simulink model "case3"  (R2024b)
settings: Solver=FixedStepAuto  StartTime=0  StopTime=1  FixedStep=1e-7  RelTol=1e-3
values from neighbouring files (symbols this model uses):
  SG_D_1_D = 0.01056    [IEEE9_case_parameters.m]    (also in case1_parameters.m; case2_parameters.m; case3_parameters.m; case4_parameters.m)
  SG_D_1_EnableSaturation = 0    [IEEE9_case_parameters.m]    (also in case1_parameters.m; case2_parameters.m; case3_parameters.m; case4_parameters.m)
  SG_D_1_f0 = 60    [IEEE9_case_parameters.m]    (also in case1_parameters.m; case2_parameters.m; case3_parameters.m; case4_parameters.m)
  SG_D_1_H = 7.5    [IEEE9_case_parameters.m]    (also in case1_parameters.m; case2_parameters.m; case3_parameters.m; case4_parameters.m)
  SG_D_1_K_A = 20    [IEEE9_case_parameters.m]    (also in case1_parameters.m; case2_parameters.m; case3_parameters.m; case4_parameters.m)
  SG_D_1_K_E = 1.000000e+1    (= 10)    [IEEE9_case_parameters.m]    (also in case1_parameters.m; case2_parameters.m; case3_parameters.m; case4_parameters.m)
  SG_D_1_K_F = 2.363    [IEEE9_case_parameters.m]    (also in case1_parameters.m; case2_parameters.m; case3_parameters.m; case4_parameters.m)
  SG_D_1_K_s = 0.5    [IEEE9_case_parameters.m]    (also in case1_parameters.m = 5; case2_parameters.m = 5; case3_parameters.m = 5; case4_parameters.m = 5)
  SG_D_1_R_a = 0.001088    [IEEE9_case_parameters.m]    (also in case1_parameters.m; case2_parameters.m; case3_parameters.m; case4_parameters.m)
  SG_D_1_S_A = 1    [IEEE9_case_parameters.m]    (also in case1_parameters.m; case2_parameters.m; case3_parameters.m; case4_parameters.m)
  SG_D_1_S_B = 0.103    [IEEE9_case_parameters.m]    (also in case1_parameters.m; case2_parameters.m; case3_parameters.m; case4_parameters.m)
  SG_D_1_S_N = 10.659857    [IEEE9_case_parameters.m]    (also in case1_parameters.m; case2_parameters.m; case3_parameters.m; case4_parameters.m)
  SG_D_1_SpeedPara = 200    [IEEE9_case_parameters.m]    (also in case1_parameters.m; case2_parameters.m; case3_parameters.m; case4_parameters.m)
  SG_D_1_T_0 = 0.720173    [IEEE9_case_parameters.m]    (also in case1_parameters.m = 0.755522; case2_parameters.m = 0.808931; case3_parameters.m = 0.869402; case4_parameters.m = 0.729316)
  SG_D_1_T_1 = 0.3    [IEEE9_case_parameters.m]    (also in case1_parameters.m; case2_parameters.m; case3_parameters.m; case4_parameters.m)
  SG_D_1_T_2 = 0.05    [IEEE9_case_parameters.m]    (also in case1_parameters.m; case2_parameters.m; case3_parameters.m; case4_parameters.m)
  SG_D_1_T_3 = 0.02    [IEEE9_case_parameters.m]    (also in case1_parameters.m; case2_parameters.m; case3_parameters.m; case4_parameters.m)
  SG_D_1_T_4 = 0.005    [IEEE9_case_parameters.m]    (also in case1_parameters.m; case2_parameters.m; case3_parameters.m; case4_parameters.m)
  SG_D_1_T_A = 0.02    [IEEE9_case_parameters.m]    (also in case1_parameters.m; case2_parameters.m; case3_parameters.m; case4_parameters.m)
  SG_D_1_T_dd = 8.000000e+0    (= 8)    [IEEE9_case_parameters.m]    (also in case1_parameters.m; case2_parameters.m; case3_parameters.m; case4_parameters.m)
  SG_D_1_T_ddd = 0.04    [IEEE9_case_parameters.m]    (also in case1_parameters.m; case2_parameters.m; case3_parameters.m; case4_parameters.m)
  SG_D_1_T_E = 0.314    [IEEE9_case_parameters.m]    (also in case1_parameters.m; case2_parameters.m; case3_parameters.m; case4_parameters.m)
  SG_D_1_T_F = 0.35    [IEEE9_case_parameters.m]    (also in case1_parameters.m; case2_parameters.m; case3_parameters.m; case4_parameters.m)
  SG_D_1_T_qd = 0.8    [IEEE9_case_parameters.m]    (also in case1_parameters.m; case2_parameters.m; case3_parameters.m; case4_parameters.m)
  SG_D_1_T_qdd = 0.02    [IEEE9_case_parameters.m]    (also in case1_parameters.m; case2_parameters.m; case3_parameters.m; case4_parameters.m)
  SG_D_1_T_speed = 0.1    [IEEE9_case_parameters.m]    (also in case1_parameters.m = 200; case2_parameters.m = 200; case3_parameters.m = 200; case4_parameters.m = 200)
  SG_D_1_T_w = 0.5    [IEEE9_case_parameters.m]    (also in case1_parameters.m; case2_parameters.m; case3_parameters.m; case4_parameters.m)
  SG_D_1_V_ref = 1.990276    [IEEE9_case_parameters.m]    (also in case1_parameters.m = 2.042296; case2_parameters.m = 2.051388; case3_parameters.m = 2.089584; case4_parameters.m = 2.01845)
  SG_D_1_w_ref = 376.991118    [IEEE9_case_parameters.m]    (also in case1_parameters.m; case2_parameters.m; case3_parameters.m; case4_parameters.m)
  SG_D_1_wb = 6.000000e+1    (= 60)    [IEEE9_case_parameters.m]    (also in case1_parameters.m; case2_parameters.m; case3_parameters.m; case4_parameters.m)
  SG_D_1_x_d = 1.9    [IEEE9_case_parameters.m]    (also in case1_parameters.m; case2_parameters.m; case3_parameters.m; case4_parameters.m)
  SG_D_1_x_dd = 0.302    [IEEE9_case_parameters.m]    (also in case1_parameters.m; case2_parameters.m; case3_parameters.m; case4_parameters.m)
  SG_D_1_x_ddd = 0.204    [IEEE9_case_parameters.m]    (also in case1_parameters.m; case2_parameters.m; case3_parameters.m; case4_parameters.m)
  SG_D_1_x_l = 0.05    [IEEE9_case_parameters.m]    (also in case1_parameters.m; case2_parameters.m; case3_parameters.m; case4_parameters.m)
  SG_D_1_x_q = 1.3    [IEEE9_case_parameters.m]    (also in case1_parameters.m; case2_parameters.m; case3_parameters.m; case4_parameters.m)
  SG_D_1_x_qd = 0.5    [IEEE9_case_parameters.m]    (also in case1_parameters.m; case2_parameters.m; case3_parameters.m; case4_parameters.m)
  SG_D_1_x_qdd = 0.3    [IEEE9_case_parameters.m]    (also in case1_parameters.m; case2_parameters.m; case3_parameters.m; case4_parameters.m)
  SG_D_2_D = 0.02    [IEEE9_case_parameters.m]    (also in case1_parameters.m; case2_parameters.m; case3_parameters.m; case4_parameters.m)
  SG_D_2_EnableSaturation = 0    [IEEE9_case_parameters.m]    (also in case1_parameters.m; case2_parameters.m; case3_parameters.m; case4_parameters.m)
  SG_D_2_f0 = 60    [IEEE9_case_parameters.m]    (also in case1_parameters.m; case2_parameters.m; case3_parameters.m; case4_parameters.m)
  SG_D_2_H = 8.000000e+0    (= 8)    [IEEE9_case_parameters.m]    (also in case1_parameters.m; case2_parameters.m; case3_parameters.m; case4_parameters.m)
  SG_D_2_K_A = 20    [IEEE9_case_parameters.m]    (also in case1_parameters.m; case2_parameters.m; case3_parameters.m; case4_parameters.m)
  SG_D_2_K_E = 1.000000e+1    (= 10)    [IEEE9_case_parameters.m]    (also in case1_parameters.m; case2_parameters.m; case3_parameters.m; case4_parameters.m)
  SG_D_2_K_F = 2.363    [IEEE9_case_parameters.m]    (also in case1_parameters.m; case2_parameters.m; case3_parameters.m; case4_parameters.m)
  SG_D_2_K_s = 0.5    [IEEE9_case_parameters.m]    (also in case1_parameters.m = 4; case2_parameters.m = 4; case3_parameters.m = 4; case4_parameters.m = 4)
  SG_D_2_R_a = 0.001088    [IEEE9_case_parameters.m]    (also in case1_parameters.m; case2_parameters.m; case3_parameters.m; case4_parameters.m)
  SG_D_2_S_A = 1    [IEEE9_case_parameters.m]    (also in case1_parameters.m; case2_parameters.m; case3_parameters.m; case4_parameters.m)
  SG_D_2_S_B = 0.103    [IEEE9_case_parameters.m]    (also in case1_parameters.m; case2_parameters.m; case3_parameters.m; case4_parameters.m)
  SG_D_2_S_N = 10.659857    [IEEE9_case_parameters.m]    (also in case1_parameters.m; case2_parameters.m; case3_parameters.m; case4_parameters.m)
  SG_D_2_SpeedPara = 200    [IEEE9_case_parameters.m]    (also in case1_parameters.m; case2_parameters.m; case3_parameters.m; case4_parameters.m)
  SG_D_2_T_0 = 1.632913    [IEEE9_case_parameters.m]    (also in case1_parameters.m = 1.632925; case2_parameters.m = 1.632915; case3_parameters.m = 1.632914; case4_parameters.m = 1.632927)
  SG_D_2_T_1 = 0.2    [IEEE9_case_parameters.m]    (also in case1_parameters.m; case2_parameters.m; case3_parameters.m; case4_parameters.m)
  SG_D_2_T_2 = 0.05    [IEEE9_case_parameters.m]    (also in case1_parameters.m; case2_parameters.m; case3_parameters.m; case4_parameters.m)
  SG_D_2_T_3 = 0.02    [IEEE9_case_parameters.m]    (also in case1_parameters.m; case2_parameters.m; case3_parameters.m; case4_parameters.m)
  SG_D_2_T_4 = 0.005    [IEEE9_case_parameters.m]    (also in case1_parameters.m; case2_parameters.m; case3_parameters.m; case4_parameters.m)
  SG_D_2_T_A = 0.02    [IEEE9_case_parameters.m]    (also in case1_parameters.m; case2_parameters.m; case3_parameters.m; case4_parameters.m)
  SG_D_2_T_dd = 7.9    [IEEE9_case_parameters.m]    (also in case1_parameters.m; case2_parameters.m; case3_parameters.m; case4_parameters.m)
  SG_D_2_T_ddd = 0.04    [IEEE9_case_parameters.m]    (also in case1_parameters.m; case2_parameters.m; case3_parameters.m; case4_parameters.m)
  SG_D_2_T_E = 0.314    [IEEE9_case_parameters.m]    (also in case1_parameters.m; case2_parameters.m; case3_parameters.m; case4_parameters.m)
  SG_D_2_T_F = 0.35    [IEEE9_case_parameters.m]    (also in case1_parameters.m; case2_parameters.m; case3_parameters.m; case4_parameters.m)
  SG_D_2_T_qd = 0.8    [IEEE9_case_parameters.m]    (also in case1_parameters.m; case2_parameters.m; case3_parameters.m; case4_parameters.m)
  SG_D_2_T_qdd = 0.015    [IEEE9_case_parameters.m]    (also in case1_parameters.m; case2_parameters.m; case3_parameters.m; case4_parameters.m)
  SG_D_2_T_speed = 0.1    [IEEE9_case_parameters.m]    (also in case1_parameters.m = 150; case2_parameters.m = 150; case3_parameters.m = 150; case4_parameters.m = 150)
  SG_D_2_T_w = 0.35    [IEEE9_case_parameters.m]    (also in case1_parameters.m; case2_parameters.m; case3_parameters.m; case4_parameters.m)
  SG_D_2_V_ref = 2.58547    [IEEE9_case_parameters.m]    (also in case1_parameters.m = 2.597896; case2_parameters.m = 2.587136; case3_parameters.m = 2.586042; case4_parameters.m = 2.599679)
  SG_D_2_w_ref = 376.991118    [IEEE9_case_parameters.m]    (also in case1_parameters.m; case2_parameters.m; case3_parameters.m; case4_parameters.m)
  SG_D_2_wb = 6.000000e+1    (= 60)    [IEEE9_case_parameters.m]    (also in case1_parameters.m; case2_parameters.m; case3_parameters.m; case4_parameters.m)
  SG_D_2_x_d = 1.8    [IEEE9_case_parameters.m]    (also in case1_parameters.m; case2_parameters.m; case3_parameters.m; case4_parameters.m)
  SG_D_2_x_dd = 0.302    [IEEE9_case_parameters.m]    (also in case1_parameters.m; case2_parameters.m; case3_parameters.m; case4_parameters.m)
  SG_D_2_x_ddd = 0.204    [IEEE9_case_parameters.m]    (also in case1_parameters.m; case2_parameters.m; case3_parameters.m; case4_parameters.m)
  SG_D_2_x_l = 0.05    [IEEE9_case_parameters.m]    (also in case1_parameters.m; case2_parameters.m; case3_parameters.m; case4_parameters.m)
  SG_D_2_x_q = 1.25    [IEEE9_case_parameters.m]    (also in case1_parameters.m; case2_parameters.m; case3_parameters.m; case4_parameters.m)
  SG_D_2_x_qd = 0.5    [IEEE9_case_parameters.m]    (also in case1_parameters.m; case2_parameters.m; case3_parameters.m; case4_parameters.m)
  SG_D_2_x_qdd = 0.3    [IEEE9_case_parameters.m]    (also in case1_parameters.m; case2_parameters.m; case3_parameters.m; case4_parameters.m)
  SG_D_3_D = 0.02    [IEEE9_case_parameters.m]    (also in case1_parameters.m; case2_parameters.m; case3_parameters.m; case4_parameters.m)
  SG_D_3_EnableSaturation = 0    [IEEE9_case_parameters.m]    (also in case1_parameters.m; case2_parameters.m; case3_parameters.m; case4_parameters.m)
  SG_D_3_f0 = 60    [IEEE9_case_parameters.m]    (also in case1_parameters.m; case2_parameters.m; case3_parameters.m; case4_parameters.m)
  SG_D_3_H = 7.7    [IEEE9_case_parameters.m]    (also in case1_parameters.m; case2_parameters.m; case3_parameters.m; case4_parameters.m)
  SG_D_3_K_A = 20    [IEEE9_case_parameters.m]    (also in case1_parameters.m; case2_parameters.m; case3_parameters.m; case4_parameters.m)
  SG_D_3_K_E = 1.000000e+1    (= 10)    [IEEE9_case_parameters.m]    (also in case1_parameters.m; case2_parameters.m; case3_parameters.m; case4_parameters.m)
  SG_D_3_K_F = 2.363    [IEEE9_case_parameters.m]    (also in case1_parameters.m; case2_parameters.m; case3_parameters.m; case4_parameters.m)
  SG_D_3_K_s = 0.2    [IEEE9_case_parameters.m]    (also in case1_parameters.m = 2; case2_parameters.m = 2; case3_parameters.m = 2; case4_parameters.m = 2)
  SG_D_3_R_a = 0.001088    [IEEE9_case_parameters.m]    (also in case1_parameters.m; case2_parameters.m; case3_parameters.m; case4_parameters.m)
  SG_D_3_S_A = 1    [IEEE9_case_parameters.m]    (also in case1_parameters.m; case2_parameters.m; case3_parameters.m; case4_parameters.m)
  SG_D_3_S_B = 0.103    [IEEE9_case_parameters.m]    (also in case1_parameters.m; case2_parameters.m; case3_parameters.m; case4_parameters.m)
  SG_D_3_S_N = 10.659857    [IEEE9_case_parameters.m]    (also in case1_parameters.m; case2_parameters.m; case3_parameters.m; case4_parameters.m)
  SG_D_3_SpeedPara = 200    [IEEE9_case_parameters.m]    (also in case1_parameters.m; case2_parameters.m; case3_parameters.m; case4_parameters.m)
  SG_D_3_T_0 = 0.850788    [IEEE9_case_parameters.m]    (also in case1_parameters.m = 0.850786; case2_parameters.m = 0.850787; case3_parameters.m; case4_parameters.m = 0.850786)
  SG_D_3_T_1 = 0.2    [IEEE9_case_parameters.m]    (also in case1_parameters.m; case2_parameters.m; case3_parameters.m; case4_parameters.m)
  SG_D_3_T_2 = 0.05    [IEEE9_case_parameters.m]    (also in case1_parameters.m; case2_parameters.m; case3_parameters.m; case4_parameters.m)
  SG_D_3_T_3 = 0.02    [IEEE9_case_parameters.m]    (also in case1_parameters.m; case2_parameters.m; case3_parameters.m; case4_parameters.m)
  SG_D_3_T_4 = 0.005    [IEEE9_case_parameters.m]    (also in case1_parameters.m; case2_parameters.m; case3_parameters.m; case4_parameters.m)
  SG_D_3_T_A = 0.02    [IEEE9_case_parameters.m]    (also in case1_parameters.m; case2_parameters.m; case3_parameters.m; case4_parameters.m)
  SG_D_3_T_dd = 8.1    [IEEE9_case_parameters.m]    (also in case1_parameters.m; case2_parameters.m; case3_parameters.m; case4_parameters.m)
  SG_D_3_T_ddd = 0.04    [IEEE9_case_parameters.m]    (also in case1_parameters.m; case2_parameters.m; case3_parameters.m; case4_parameters.m)
  SG_D_3_T_E = 0.314    [IEEE9_case_parameters.m]    (also in case1_parameters.m; case2_parameters.m; case3_parameters.m; case4_parameters.m)
  SG_D_3_T_F = 0.35    [IEEE9_case_parameters.m]    (also in case1_parameters.m; case2_parameters.m; case3_parameters.m; case4_parameters.m)
  SG_D_3_T_qd = 0.8    [IEEE9_case_parameters.m]    (also in case1_parameters.m; case2_parameters.m; case3_parameters.m; case4_parameters.m)
  SG_D_3_T_qdd = 0.015    [IEEE9_case_parameters.m]    (also in case1_parameters.m; case2_parameters.m; case3_parameters.m; case4_parameters.m)
  SG_D_3_T_speed = 0.1    [IEEE9_case_parameters.m]    (also in case1_parameters.m = 180; case2_parameters.m = 180; case3_parameters.m = 180; case4_parameters.m = 180)
  SG_D_3_T_w = 0.4    [IEEE9_case_parameters.m]    (also in case1_parameters.m; case2_parameters.m; case3_parameters.m; case4_parameters.m)
  SG_D_3_V_ref = 1.892727    [IEEE9_case_parameters.m]    (also in case1_parameters.m = 1.906439; case2_parameters.m = 1.895535; case3_parameters.m = 1.892105; case4_parameters.m = 1.906598)
  SG_D_3_w_ref = 376.991118    [IEEE9_case_parameters.m]    (also in case1_parameters.m; case2_parameters.m; case3_parameters.m; case4_parameters.m)
  SG_D_3_wb = 6.000000e+1    (= 60)    [IEEE9_case_parameters.m]    (also in case1_parameters.m; case2_parameters.m; case3_parameters.m; case4_parameters.m)
  SG_D_3_x_d = 1.85    [IEEE9_case_parameters.m]    (also in case1_parameters.m; case2_parameters.m; case3_parameters.m; case4_parameters.m)
  SG_D_3_x_dd = 0.302    [IEEE9_case_parameters.m]    (also in case1_parameters.m; case2_parameters.m; case3_parameters.m; case4_parameters.m)
  SG_D_3_x_ddd = 0.204    [IEEE9_case_parameters.m]    (also in case1_parameters.m; case2_parameters.m; case3_parameters.m; case4_parameters.m)
  SG_D_3_x_l = 0.05    [IEEE9_case_parameters.m]    (also in case1_parameters.m; case2_parameters.m; case3_parameters.m; case4_parameters.m)
  SG_D_3_x_q = 1.2    [IEEE9_case_parameters.m]    (also in case1_parameters.m; case2_parameters.m; case3_parameters.m; case4_parameters.m)
  SG_D_3_x_qd = 0.5    [IEEE9_case_parameters.m]    (also in case1_parameters.m; case2_parameters.m; case3_parameters.m; case4_parameters.m)
  SG_D_3_x_qdd = 0.3    [IEEE9_case_parameters.m]    (also in case1_parameters.m; case2_parameters.m; case3_parameters.m; case4_parameters.m)
(part 9 of 12)

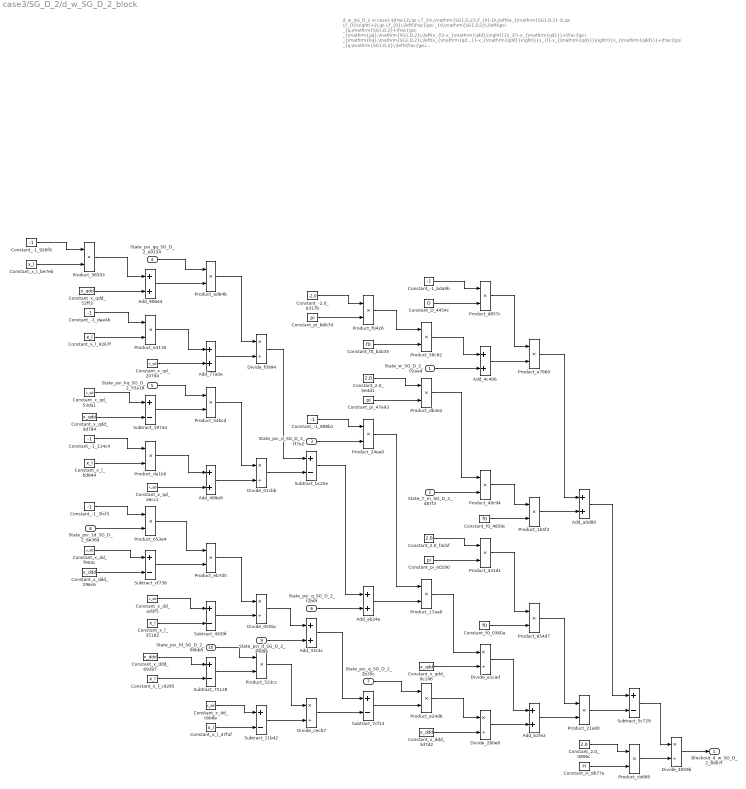
== system case3/SG_D_2/d_w_SG_D_2_block ==
  note: d_w_SG_D_2 in case3
      | $\frac{2\,\pi \,T_{m,\mathrm{SG},D,2}\,f_{0}-D\,\left(w_{\mathrm{SG},D,2}-2\,\pi \,f_{0}\right)+2\,\pi \,f_{0}\,\left(\frac{\psi _{d,\mathrm{SG},D,2}\,\left(\psi _{q,\mathrm{SG},D,2}+\frac{\psi _{\mathrm{gq},\mathrm{SG},D,2}\,\left(x_{l}-x_{\mathrm{qdd}}\right)}{x_{l}-x_{\mathrm{qd}}}+\frac{\psi _{\mathrm{kq},\mathrm{SG},D,2}\,\left(x_{\mathrm{qd}}-x_{\mathrm{qdd}}\right)}{x_{l}-x_{\mathrm{qd}}}\right)}{x_{\mathrm{qdd}}}+\frac{\psi _{q,\mathrm{SG},D,2}\,\left(\frac{\psi _{\mathrm{1d},\mathrm{SG},D,2}\,\left(x_{\mathrm{dd}}-x_{\mathrm{ddd}}\right)}{x_{\mathrm{dd}}-x_{l}}-\psi _{d,\mathrm{SG},D,2}+\frac{\psi _{\mathrm{fd},\mathrm{SG},D,2}\,\left(x_{\mathrm{ddd}}-x_{l}\right)}{x_{\mathrm{dd}}-x_{l}}\right)}{x_{\mathrm{ddd}}}\right)}{2\,H}$
      | Automatically generated on 2025-10-31 19:00:18 .
  State_w_SG_D_2_02aad : Inport
  State_T_m_SG_D_2_487f3 : Inport  Port=2
  State_psi_d_SG_D_2_ff7e2 : Inport  Port=3
  State_psi_gq_SG_D_2_e9134 : Inport  Port=4
  State_psi_kq_SG_D_2_55a18 : Inport  Port=5
  State_psi_q_SG_D_2_f2b6f : Inport  Port=6
  State_psi_q_SG_D_2_2b35c : Inport  Port=7
  State_psi_1d_SG_D_2_8e36d : Inport  Port=8
  State_psi_d_SG_D_2_34d9a : Inport  Port=9
  State_psi_fd_SG_D_2_06bb8 : Inport  Port=10
  Add_33c4c : Sum
  Add_499e9 : Sum
  Add_4c406 : Sum
  Add_77a0e : Sum
  Add_90644 : Sum
  Add_a0d80 : Sum
  Add_ab24e : Sum
  Add_b2fe2 : Sum
  Constant_-1_114c4 : Constant  Value=-1
  Constant_-1_3fcf5 : Constant  Value=-1
  Constant_-1_898b1 : Constant  Value=-1
  Constant_-1_926f9 : Constant  Value=-1
  Constant_-1_bda9b : Constant  Value=-1
  Constant_-1_dae4b : Constant  Value=-1
  Constant_-2.0_0317b : Constant  Value=-2.0
  Constant_2.0_0806c : Constant  Value=2.0
  Constant_2.0_5e4d1 : Constant  Value=2.0
  Constant_2.0_f4cbf : Constant  Value=2.0
  Constant_D_4454c : Constant  Value=D
  Constant_H_8b77e : Constant  Value=H
  Constant_f0_0360a : Constant  Value=f0
  Constant_f0_4859c : Constant  Value=f0
  Constant_f0_bab35 : Constant  Value=f0
  Constant_pi_47e93 : Constant  Value=pi
  Constant_pi_b6b7d : Constant  Value=pi
  Constant_pi_e0290 : Constant  Value=pi
  Constant_x_dd_ad3f5 : Constant  Value=x_dd
  Constant_x_dd_cbb8e : Constant  Value=x_dd
  Constant_x_dd_f954c : Constant  Value=x_dd
  Constant_x_ddd_296c6 : Constant  Value=x_ddd
  Constant_x_ddd_3d7d2 : Constant  Value=x_ddd
  Constant_x_ddd_69397 : Constant  Value=x_ddd
  Constant_x_l_35182 : Constant  Value=x_l
  Constant_x_l_47faf : Constant  Value=x_l
  Constant_x_l_9267f : Constant  Value=x_l
  Constant_x_l_bd844 : Constant  Value=x_l
  Constant_x_l_be7eb : Constant  Value=x_l
  Constant_x_l_c9295 : Constant  Value=x_l
  Constant_x_qd_20794 : Constant  Value=x_qd
  Constant_x_qd_53da1 : Constant  Value=x_qd
  Constant_x_qd_a6cc1 : Constant  Value=x_qd
  Constant_x_qdd_0c146 : Constant  Value=x_qdd
  Constant_x_qdd_0d784 : Constant  Value=x_qdd
  Constant_x_qdd_52ff3 : Constant  Value=x_qdd
  Divide_01cbb : Product  Inputs=*/
  Divide_055bc : Product  Inputs=*/
  Divide_280e8 : Product  Inputs=*/
  Divide_4059b : Product  Inputs=*/
  Divide_cecb7 : Product  Inputs=*/
  Divide_e1cad : Product  Inputs=*/
  Divide_f0994 : Product  Inputs=*/
  Product_17aa0 : Product
  Product_1b5f2 : Product
  Product_21a80 : Product
  Product_24ee0 : Product
  Product_36593 : Product
  Product_431d1 : Product
  Product_49c94 : Product
  Product_523cc : Product
  Product_54bcd : Product
  Product_58c82 : Product
  Product_653e4 : Product
  Product_854d7 : Product
  Product_ad84b : Product
  Product_cb688 : Product
  Product_d857c : Product
  Product_da1b0 : Product
  Product_db3e2 : Product
  Product_e24d6 : Product
  Product_e3130 : Product
  Product_e7869 : Product
  Product_eb7d5 : Product
  Product_f0426 : Product
  Subtract_11b42 : Sum  Inputs=+-
  Subtract_19744 : Sum  Inputs=+-
  Subtract_4939f : Sum  Inputs=+-
  Subtract_5c729 : Sum  Inputs=+-
  Subtract_75128 : Sum  Inputs=+-
  Subtract_7cf13 : Sum  Inputs=+-
  Subtract_bc25e : Sum  Inputs=+-
  Subtract_cf738 : Sum  Inputs=+-
  Blockout_d_w_SG_D_2_8967f : Outport
  wires:
  Constant_x_qd_53da1/1 -> Subtract_19744/1
  Constant_-1_114c4/1 -> Product_da1b0/1
  Constant_-1_926f9/1 -> Product_36593/1
  Constant_x_qdd_0d784/1 -> Subtract_19744/2
  Subtract_11b42/1 -> Divide_cecb7/2
  Constant_x_l_bd844/1 -> Product_da1b0/2
  Constant_x_l_be7eb/1 -> Product_36593/2
  Product_da1b0/1 -> Add_499e9/1
  Product_36593/1 -> Add_90644/1
  Constant_x_l_35182/1 -> Subtract_4939f/2
  Constant_x_l_9267f/1 -> Product_e3130/2
  Constant_x_ddd_3d7d2/1 -> Divide_280e8/2
  Subtract_75128/1 -> Product_523cc/2
  Constant_x_qd_a6cc1/1 -> Add_499e9/2
  Constant_x_qdd_52ff3/1 -> Add_90644/2
  Constant_-1_dae4b/1 -> Product_e3130/1
  State_psi_d_SG_D_2_ff7e2/1 -> Product_24ee0/2
  Constant_-1_3fcf5/1 -> Product_653e4/1
  State_w_SG_D_2_02aad/1 -> Add_4c406/2
  Product_e3130/1 -> Add_77a0e/1
  State_psi_1d_SG_D_2_8e36d/1 -> Product_653e4/2
  Constant_x_dd_f954c/1 -> Subtract_cf738/1
  Divide_f0994/1 -> Subtract_bc25e/1
  Subtract_19744/1 -> Product_54bcd/2
  Constant_x_ddd_296c6/1 -> Subtract_cf738/2
  State_psi_gq_SG_D_2_e9134/1 -> Product_ad84b/1
  Add_499e9/1 -> Divide_01cbb/2
  State_psi_d_SG_D_2_34d9a/1 -> Add_33c4c/2
  Add_90644/1 -> Product_ad84b/2
  Constant_x_qd_20794/1 -> Add_77a0e/2
  State_psi_kq_SG_D_2_55a18/1 -> Product_54bcd/1
  Product_653e4/1 -> Product_eb7d5/1
  Subtract_cf738/1 -> Product_eb7d5/2
  Constant_pi_47e93/1 -> Product_db3e2/2
  Constant_x_dd_ad3f5/1 -> Subtract_4939f/1
  Constant_x_ddd_69397/1 -> Subtract_75128/1
  Constant_x_l_c9295/1 -> Subtract_75128/2
  Product_ad84b/1 -> Divide_f0994/1
  Add_77a0e/1 -> Divide_f0994/2
  Add_ab24e/1 -> Product_17aa0/2
  Product_54bcd/1 -> Divide_01cbb/1
  Constant_pi_b6b7d/1 -> Product_f0426/2
  Product_eb7d5/1 -> Divide_055bc/1
  Subtract_4939f/1 -> Divide_055bc/2
  State_psi_fd_SG_D_2_06bb8/1 -> Product_523cc/1
  Divide_055bc/1 -> Add_33c4c/1
  Constant_x_dd_cbb8e/1 -> Subtract_11b42/1
  Constant_x_l_47faf/1 -> Subtract_11b42/2
  Divide_01cbb/1 -> Subtract_bc25e/2
  Product_523cc/1 -> Divide_cecb7/1
  Constant_-1_898b1/1 -> Product_24ee0/1
  Constant_-2.0_0317b/1 -> Product_f0426/1
  Subtract_bc25e/1 -> Add_ab24e/1
  Subtract_7cf13/1 -> Product_e24d6/2
  State_psi_q_SG_D_2_f2b6f/1 -> Add_ab24e/2
  Constant_D_4454c/1 -> Product_d857c/2
  Add_33c4c/1 -> Subtract_7cf13/1
  Divide_cecb7/1 -> Subtract_7cf13/2
  Product_f0426/1 -> Product_58c82/1
  Constant_f0_bab35/1 -> Product_58c82/2
  Constant_2.0_5e4d1/1 -> Product_db3e2/1
  Product_24ee0/1 -> Product_17aa0/1
  State_psi_q_SG_D_2_2b35c/1 -> Product_e24d6/1
  Constant_-1_bda9b/1 -> Product_d857c/1
  Product_58c82/1 -> Add_4c406/1
  Product_db3e2/1 -> Product_49c94/1
  State_T_m_SG_D_2_487f3/1 -> Product_49c94/2
  Constant_2.0_f4cbf/1 -> Product_431d1/1
  Constant_pi_e0290/1 -> Product_431d1/2
  Product_17aa0/1 -> Divide_e1cad/1
  Constant_x_qdd_0c146/1 -> Divide_e1cad/2
  Product_e24d6/1 -> Divide_280e8/1
  Product_d857c/1 -> Product_e7869/1
  Add_4c406/1 -> Product_e7869/2
  Product_49c94/1 -> Product_1b5f2/1
  Constant_f0_4859c/1 -> Product_1b5f2/2
  Product_431d1/1 -> Product_854d7/1
  Constant_f0_0360a/1 -> Product_854d7/2
  Divide_e1cad/1 -> Add_b2fe2/1
  Divide_280e8/1 -> Add_b2fe2/2
  Product_e7869/1 -> Add_a0d80/1
  Product_1b5f2/1 -> Add_a0d80/2
  Product_854d7/1 -> Product_21a80/1
  Add_b2fe2/1 -> Product_21a80/2
  Add_a0d80/1 -> Subtract_5c729/1
  Product_21a80/1 -> Subtract_5c729/2
  Constant_2.0_0806c/1 -> Product_cb688/1
  Constant_H_8b77e/1 -> Product_cb688/2
  Subtract_5c729/1 -> Divide_4059b/1
  Product_cb688/1 -> Divide_4059b/2
  Divide_4059b/1 -> Blockout_d_w_SG_D_2_8967f/1

== system case3/SG_D_2/i_d_SG_D_2_block ==
  note: i_d_SG_D_2 in case3
      | $\frac{\sin\left(\theta _{\mathrm{SG},D,2}\right)\,\left(\frac{\psi _{\mathrm{1d},\mathrm{SG},D,2}\,\left(x_{\mathrm{dd}}-x_{\mathrm{ddd}}\right)}{x_{\mathrm{dd}}-x_{l}}-\psi _{d,\mathrm{SG},D,2}+\frac{\psi _{\mathrm{fd},\mathrm{SG},D,2}\,\left(x_{\mathrm{ddd}}-x_{l}\right)}{x_{\mathrm{dd}}-x_{l}}\right)}{x_{\mathrm{ddd}}}-\frac{\cos\left(\theta _{\mathrm{SG},D,2}\right)\,\left(\psi _{q,\mathrm{SG},D,2}+\frac{\psi _{\mathrm{gq},\mathrm{SG},D,2}\,\left(x_{l}-x_{\mathrm{qdd}}\right)}{x_{l}-x_{\mathrm{qd}}}+\frac{\psi _{\mathrm{kq},\mathrm{SG},D,2}\,\left(x_{\mathrm{qd}}-x_{\mathrm{qdd}}\right)}{x_{l}-x_{\mathrm{qd}}}\right)}{x_{\mathrm{qdd}}}$
      | Automatically generated on 2025-10-31 19:00:34 .
  State_psi_gq_SG_D_2_2ee45 : Inport
  State_psi_kq_SG_D_2_8f947 : Inport  Port=2
  State_psi_q_SG_D_2_858f7 : Inport  Port=3
  State_theta_SG_D_2_26ddd : Inport  Port=4
  State_psi_1d_SG_D_2_56a6d : Inport  Port=5
  State_psi_d_SG_D_2_e3a72 : Inport  Port=6
  State_psi_fd_SG_D_2_d0a13 : Inport  Port=7
  State_theta_SG_D_2_96e4e : Inport  Port=8
  Add_15c2d : Sum
  Add_99f96 : Sum
  Add_9b9a9 : Sum
  Add_d13ea : Sum
  Add_d6754 : Sum
  Constant_-1_01e66 : Constant  Value=-1
  Constant_-1_353f5 : Constant  Value=-1
  Constant_-1_69baf : Constant  Value=-1
  Constant_-1_ad66e : Constant  Value=-1
  Constant_-1_d99b1 : Constant  Value=-1
  Constant_x_dd_93d65 : Constant  Value=x_dd
  Constant_x_dd_e7ec5 : Constant  Value=x_dd
  Constant_x_dd_ec87c : Constant  Value=x_dd
  Constant_x_ddd_3e8db : Constant  Value=x_ddd
  Constant_x_ddd_e6e80 : Constant  Value=x_ddd
  Constant_x_ddd_fb939 : Constant  Value=x_ddd
  Constant_x_l_1d95e : Constant  Value=x_l
  Constant_x_l_4d988 : Constant  Value=x_l
  Constant_x_l_51fa7 : Constant  Value=x_l
  Constant_x_l_64c65 : Constant  Value=x_l
  Constant_x_l_8ce22 : Constant  Value=x_l
  Constant_x_l_ca406 : Constant  Value=x_l
  Constant_x_qd_b7bde : Constant  Value=x_qd
  Constant_x_qd_c4f16 : Constant  Value=x_qd
  Constant_x_qd_e8a99 : Constant  Value=x_qd
  Constant_x_qdd_3ac4e : Constant  Value=x_qdd
  Constant_x_qdd_7bf30 : Constant  Value=x_qdd
  Constant_x_qdd_ffc10 : Constant  Value=x_qdd
  Divide_132b9 : Product  Inputs=*/
  Divide_879d2 : Product  Inputs=*/
  Divide_992c4 : Product  Inputs=*/
  Divide_aaead : Product  Inputs=*/
  Divide_afcde : Product  Inputs=*/
  Divide_c19bf : Product  Inputs=*/
  MathFunc_cos_aa71b : Trigonometry  Operator=cos
  MathFunc_sin_46ac6 : Trigonometry
  Product_13234 : Product
  Product_52cd7 : Product
  Product_66707 : Product
  Product_84f8a : Product
  Product_9011d : Product
  Product_93471 : Product
  Product_afed6 : Product
  Product_b69c8 : Product
  Product_ce9d6 : Product
  Product_f0647 : Product
  Product_f9d19 : Product
  Subtract_0f100 : Sum  Inputs=+-
  Subtract_1d93c : Sum  Inputs=+-
  Subtract_499a0 : Sum  Inputs=+-
  Subtract_79531 : Sum  Inputs=+-
  Subtract_85321 : Sum  Inputs=+-
  Subtract_91b38 : Sum  Inputs=+-
  Subtract_d4dae : Sum  Inputs=+-
  Subtract_d676a : Sum  Inputs=+-
  Blockout_i_d_SG_D_2_b1c5f : Outport
  wires:
  Constant_x_ddd_3e8db/1 -> Subtract_499a0/1
  Constant_x_qd_e8a99/1 -> Subtract_79531/1
  Constant_-1_d99b1/1 -> Product_f9d19/1
  Constant_-1_353f5/1 -> Product_f0647/1
  Subtract_0f100/1 -> Blockout_i_d_SG_D_2_b1c5f/1
  Constant_x_qdd_ffc10/1 -> Subtract_79531/2
  Constant_x_l_64c65/1 -> Product_f9d19/2
  Constant_x_l_51fa7/1 -> Product_f0647/2
  Product_f9d19/1 -> Add_d13ea/1
  Product_f0647/1 -> Add_99f96/1
  Constant_x_l_8ce22/1 -> Product_66707/2
  Constant_x_qd_b7bde/1 -> Add_d13ea/2
  Constant_x_qdd_3ac4e/1 -> Add_99f96/2
  Constant_x_qdd_7bf30/1 -> Divide_132b9/2
  MathFunc_cos_aa71b/1 -> Product_93471/2
  Constant_-1_69baf/1 -> Product_66707/1
  State_psi_gq_SG_D_2_2ee45/1 -> Product_9011d/1
  Subtract_499a0/1 -> Product_afed6/2
  Product_13234/1 -> Product_ce9d6/1
  Add_d13ea/1 -> Divide_992c4/2
  Add_99f96/1 -> Product_9011d/2
  Product_afed6/1 -> Divide_afcde/1
  Product_66707/1 -> Add_d6754/1
  Constant_x_qd_c4f16/1 -> Add_d6754/2
  State_theta_SG_D_2_96e4e/1 -> MathFunc_sin_46ac6/1
  State_psi_kq_SG_D_2_8f947/1 -> Product_84f8a/1
  Add_15c2d/1 -> Subtract_1d93c/1
  Subtract_79531/1 -> Product_84f8a/2
  Product_9011d/1 -> Divide_aaead/1
  Constant_-1_01e66/1 -> Product_13234/1
  State_psi_1d_SG_D_2_56a6d/1 -> Product_13234/2
  State_psi_fd_SG_D_2_d0a13/1 -> Product_afed6/1
  Constant_x_dd_ec87c/1 -> Subtract_d4dae/1
  Product_ce9d6/1 -> Divide_c19bf/1
  Constant_x_ddd_e6e80/1 -> Subtract_d4dae/2
  Divide_afcde/1 -> Subtract_1d93c/2
  Add_d6754/1 -> Divide_aaead/2
  Product_b69c8/1 -> Divide_879d2/1
  Product_84f8a/1 -> Divide_992c4/1
  Constant_-1_ad66e/1 -> Product_52cd7/1
  Subtract_d676a/1 -> Divide_afcde/2
  Subtract_d4dae/1 -> Product_ce9d6/2
  Constant_x_dd_93d65/1 -> Subtract_85321/1
  Subtract_1d93c/1 -> Product_b69c8/1
  Constant_x_l_4d988/1 -> Subtract_85321/2
  Constant_x_l_ca406/1 -> Subtract_499a0/2
  Divide_aaead/1 -> Subtract_91b38/1
  Divide_879d2/1 -> Subtract_0f100/2
  Divide_992c4/1 -> Subtract_91b38/2
  Subtract_85321/1 -> Divide_c19bf/2
  Constant_x_dd_e7ec5/1 -> Subtract_d676a/1
  Divide_132b9/1 -> Subtract_0f100/1
  Constant_x_l_1d95e/1 -> Subtract_d676a/2
  Subtract_91b38/1 -> Add_9b9a9/1
  State_psi_q_SG_D_2_858f7/1 -> Add_9b9a9/2
  Constant_x_ddd_fb939/1 -> Divide_879d2/2
  MathFunc_sin_46ac6/1 -> Product_b69c8/2
  Divide_c19bf/1 -> Add_15c2d/1
  State_psi_d_SG_D_2_e3a72/1 -> Add_15c2d/2
  Add_9b9a9/1 -> Product_52cd7/2
  State_theta_SG_D_2_26ddd/1 -> MathFunc_cos_aa71b/1
  Product_52cd7/1 -> Product_93471/1
  Product_93471/1 -> Divide_132b9/1

== system case3/SG_D_2/i_q_SG_D_2_block ==
  note: i_q_SG_D_2 in case3
      | $-\frac{\sin\left(\theta _{\mathrm{SG},D,2}\right)\,\left(\psi _{q,\mathrm{SG},D,2}+\frac{\psi _{\mathrm{gq},\mathrm{SG},D,2}\,\left(x_{l}-x_{\mathrm{qdd}}\right)}{x_{l}-x_{\mathrm{qd}}}+\frac{\psi _{\mathrm{kq},\mathrm{SG},D,2}\,\left(x_{\mathrm{qd}}-x_{\mathrm{qdd}}\right)}{x_{l}-x_{\mathrm{qd}}}\right)}{x_{\mathrm{qdd}}}-\frac{\cos\left(\theta _{\mathrm{SG},D,2}\right)\,\left(\frac{\psi _{\mathrm{1d},\mathrm{SG},D,2}\,\left(x_{\mathrm{dd}}-x_{\mathrm{ddd}}\right)}{x_{\mathrm{dd}}-x_{l}}-\psi _{d,\mathrm{SG},D,2}+\frac{\psi _{\mathrm{fd},\mathrm{SG},D,2}\,\left(x_{\mathrm{ddd}}-x_{l}\right)}{x_{\mathrm{dd}}-x_{l}}\right)}{x_{\mathrm{ddd}}}$
      | Automatically generated on 2025-10-31 19:00:38 .
  State_psi_gq_SG_D_2_7b19c : Inport
  State_psi_kq_SG_D_2_0c2bc : Inport  Port=2
  State_psi_q_SG_D_2_1cc4f : Inport  Port=3
  State_theta_SG_D_2_75646 : Inport  Port=4
  State_psi_1d_SG_D_2_4f110 : Inport  Port=5
  State_psi_d_SG_D_2_a879f : Inport  Port=6
  State_psi_fd_SG_D_2_1b685 : Inport  Port=7
  State_theta_SG_D_2_3ab4c : Inport  Port=8
  Add_192b0 : Sum
  Add_4b84a : Sum
  Add_58b7d : Sum
  Add_5da11 : Sum
  Add_632e0 : Sum
  Add_bbeb3 : Sum
  Constant_-1_0dda3 : Constant  Value=-1
  Constant_-1_0f492 : Constant  Value=-1
  Constant_-1_104ba : Constant  Value=-1
  Constant_-1_2d780 : Constant  Value=-1
  Constant_-1_adec8 : Constant  Value=-1
  Constant_x_dd_3529d : Constant  Value=x_dd
  Constant_x_dd_753ef : Constant  Value=x_dd
  Constant_x_dd_a060d : Constant  Value=x_dd
  Constant_x_ddd_b66f1 : Constant  Value=x_ddd
  Constant_x_ddd_c45ff : Constant  Value=x_ddd
  Constant_x_ddd_f1c79 : Constant  Value=x_ddd
  Constant_x_l_01da5 : Constant  Value=x_l
  Constant_x_l_24667 : Constant  Value=x_l
  Constant_x_l_4df82 : Constant  Value=x_l
  Constant_x_l_59496 : Constant  Value=x_l
  Constant_x_l_6302b : Constant  Value=x_l
  Constant_x_l_d5bd7 : Constant  Value=x_l
  Constant_x_qd_a417e : Constant  Value=x_qd
  Constant_x_qd_b1182 : Constant  Value=x_qd
  Constant_x_qd_c8077 : Constant  Value=x_qd
  Constant_x_qdd_03e38 : Constant  Value=x_qdd
  Constant_x_qdd_62954 : Constant  Value=x_qdd
  Constant_x_qdd_7d781 : Constant  Value=x_qdd
  Divide_06387 : Product  Inputs=*/
  Divide_0e3e6 : Product  Inputs=*/
  Divide_2008a : Product  Inputs=*/
  Divide_657f8 : Product  Inputs=*/
  Divide_6aab6 : Product  Inputs=*/
  Divide_fed1e : Product  Inputs=*/
  MathFunc_cos_2a8e1 : Trigonometry  Operator=cos
  MathFunc_sin_e5e71 : Trigonometry
  Product_482b0 : Product
  Product_5b3ff : Product
  Product_688eb : Product
  Product_7e174 : Product
  Product_8dc67 : Product
  Product_be859 : Product
  Product_c45aa : Product
  Product_d2b17 : Product
  Product_dadf9 : Product
  Product_dcbad : Product
  Product_eedae : Product
  Subtract_30d78 : Sum  Inputs=+-
  Subtract_3d93c : Sum  Inputs=+-
  Subtract_45209 : Sum  Inputs=+-
  Subtract_85b57 : Sum  Inputs=+-
  Subtract_bd56a : Sum  Inputs=+-
  Subtract_e1f7c : Sum  Inputs=+-
  Subtract_ef54d : Sum  Inputs=+-
  Blockout_i_q_SG_D_2_91d2d : Outport
  wires:
  MathFunc_sin_e5e71/1 -> Product_dcbad/2
  Product_8dc67/1 -> Product_dcbad/1
  Constant_-1_0f492/1 -> Product_688eb/1
  Constant_-1_adec8/1 -> Product_482b0/1
  Constant_x_l_01da5/1 -> Product_688eb/2
  Product_688eb/1 -> Add_bbeb3/1
  Subtract_45209/1 -> Product_5b3ff/2
  Constant_x_qdd_62954/1 -> Subtract_bd56a/2
  Constant_x_qdd_03e38/1 -> Add_bbeb3/2
  Add_4b84a/1 -> Product_8dc67/2
  Constant_x_l_d5bd7/1 -> Product_482b0/2
  Constant_x_qd_a417e/1 -> Subtract_bd56a/1
  Constant_-1_2d780/1 -> Product_be859/1
  Constant_x_l_6302b/1 -> Product_be859/2
  State_psi_1d_SG_D_2_4f110/1 -> Product_7e174/2
  State_psi_gq_SG_D_2_7b19c/1 -> Product_d2b17/1
  Add_bbeb3/1 -> Product_d2b17/2
  Product_482b0/1 -> Add_632e0/1
  Divide_06387/1 -> Add_192b0/1
  Constant_x_qd_c8077/1 -> Add_632e0/2
  State_psi_kq_SG_D_2_0c2bc/1 -> Product_c45aa/1
  Add_5da11/1 -> Subtract_3d93c/1
  Constant_x_ddd_f1c79/1 -> Subtract_45209/2
  Subtract_bd56a/1 -> Product_c45aa/2
  Product_be859/1 -> Add_58b7d/1
  Constant_x_qd_b1182/1 -> Add_58b7d/2
  Constant_-1_0dda3/1 -> Product_7e174/1
  Constant_x_l_59496/1 -> Subtract_e1f7c/2
  Constant_x_dd_a060d/1 -> Subtract_45209/1
  Product_d2b17/1 -> Divide_657f8/1
  Divide_2008a/1 -> Subtract_3d93c/2
  Add_632e0/1 -> Divide_657f8/2
  Product_eedae/1 -> Divide_0e3e6/1
  Product_c45aa/1 -> Divide_6aab6/1
  Constant_-1_104ba/1 -> Product_8dc67/1
  Product_7e174/1 -> Product_5b3ff/1
  Add_58b7d/1 -> Divide_6aab6/2
  Constant_x_dd_3529d/1 -> Subtract_85b57/1
  Subtract_3d93c/1 -> Product_eedae/1
  Subtract_ef54d/1 -> Product_dadf9/2
  Constant_x_l_4df82/1 -> Subtract_85b57/2
  Constant_x_ddd_b66f1/1 -> Subtract_ef54d/1
  Constant_x_l_24667/1 -> Subtract_ef54d/2
  Divide_657f8/1 -> Subtract_30d78/1
  Divide_0e3e6/1 -> Add_192b0/2
  Product_dadf9/1 -> Divide_2008a/1
  Divide_6aab6/1 -> Subtract_30d78/2
  Subtract_e1f7c/1 -> Divide_2008a/2
  Product_5b3ff/1 -> Divide_fed1e/1
  Subtract_85b57/1 -> Divide_fed1e/2
  Constant_x_qdd_7d781/1 -> Divide_06387/2
  State_psi_fd_SG_D_2_1b685/1 -> Product_dadf9/1
  Constant_x_dd_753ef/1 -> Subtract_e1f7c/1
  Subtract_30d78/1 -> Add_4b84a/1
  State_psi_q_SG_D_2_1cc4f/1 -> Add_4b84a/2
  Constant_x_ddd_c45ff/1 -> Divide_0e3e6/2
  Divide_fed1e/1 -> Add_5da11/1
  State_psi_d_SG_D_2_a879f/1 -> Add_5da11/2
  State_theta_SG_D_2_75646/1 -> MathFunc_sin_e5e71/1
  State_theta_SG_D_2_3ab4c/1 -> MathFunc_cos_2a8e1/1
  MathFunc_cos_2a8e1/1 -> Product_eedae/2
  Product_dcbad/1 -> Divide_06387/1
  Add_192b0/1 -> Blockout_i_q_SG_D_2_91d2d/1

== system case3/SG_D_2/theta_SG_D_2_out_block ==
  note: theta_SG_D_2_out in case3
      | $\theta _{\mathrm{SG},D,2}$
      | Automatically generated on 2025-10-31 19:00:43 .
  State_theta_SG_D_2_c18fe : Inport
  Blockout_theta_SG_D_2_out_3c0c9 : Outport
  wires:
  State_theta_SG_D_2_c18fe/1 -> Blockout_theta_SG_D_2_out_3c0c9/1

== system case3/SG_D_2/w_SG_D_2_out_block ==
  note: w_SG_D_2_out in case3
      | $w_{\mathrm{SG},D,2}$
      | Automatically generated on 2025-10-31 19:00:42 .
  State_w_SG_D_2_ed650 : Inport
  Blockout_w_SG_D_2_out_9b37d : Outport
  wires:
  State_w_SG_D_2_ed650/1 -> Blockout_w_SG_D_2_out_9b37d/1

== system case3/SG_D_3/T_e_SG_D_3_block ==
  note: T_e_SG_D_3 in case3
      | $-\frac{\psi _{d,\mathrm{SG},D,3}\,\left(\psi _{q,\mathrm{SG},D,3}+\frac{\psi _{\mathrm{gq},\mathrm{SG},D,3}\,\left(x_{l}-x_{\mathrm{qdd}}\right)}{x_{l}-x_{\mathrm{qd}}}+\frac{\psi _{\mathrm{kq},\mathrm{SG},D,3}\,\left(x_{\mathrm{qd}}-x_{\mathrm{qdd}}\right)}{x_{l}-x_{\mathrm{qd}}}\right)}{x_{\mathrm{qdd}}}-\frac{\psi _{q,\mathrm{SG},D,3}\,\left(\frac{\psi _{\mathrm{1d},\mathrm{SG},D,3}\,\left(x_{\mathrm{dd}}-x_{\mathrm{ddd}}\right)}{x_{\mathrm{dd}}-x_{l}}-\psi _{d,\mathrm{SG},D,3}+\frac{\psi _{\mathrm{fd},\mathrm{SG},D,3}\,\left(x_{\mathrm{ddd}}-x_{l}\right)}{x_{\mathrm{dd}}-x_{l}}\right)}{x_{\mathrm{ddd}}}$
      | Automatically generated on 2025-10-31 19:01:42 .
  State_psi_d_SG_D_3_1c144 : Inport
  State_psi_gq_SG_D_3_42e3f : Inport  Port=2
  State_psi_kq_SG_D_3_2048a : Inport  Port=3
  State_psi_q_SG_D_3_76dcc : Inport  Port=4
  State_psi_q_SG_D_3_c10b9 : Inport  Port=5
  State_psi_1d_SG_D_3_ba052 : Inport  Port=6
  State_psi_d_SG_D_3_65d7f : Inport  Port=7
  State_psi_fd_SG_D_3_c97e9 : Inport  Port=8
  Add_0f122 : Sum
  Add_1f3c8 : Sum
  Add_39479 : Sum
  Add_41f88 : Sum
  Add_42a7e : Sum
  Add_84477 : Sum
  Constant_-1_0749c : Constant  Value=-1
  Constant_-1_25f76 : Constant  Value=-1
  Constant_-1_47889 : Constant  Value=-1
  Constant_-1_bd1df : Constant  Value=-1
  Constant_-1_d378a : Constant  Value=-1
  Constant_x_dd_4d15d : Constant  Value=x_dd
  Constant_x_dd_dddf6 : Constant  Value=x_dd
  Constant_x_dd_fdaa2 : Constant  Value=x_dd
  Constant_x_ddd_39604 : Constant  Value=x_ddd
  Constant_x_ddd_592bf : Constant  Value=x_ddd
  Constant_x_ddd_e3129 : Constant  Value=x_ddd
  Constant_x_l_086ea : Constant  Value=x_l
  Constant_x_l_08ff2 : Constant  Value=x_l
  Constant_x_l_26133 : Constant  Value=x_l
  Constant_x_l_6d679 : Constant  Value=x_l
  Constant_x_l_b235b : Constant  Value=x_l
  Constant_x_l_bb8da : Constant  Value=x_l
  Constant_x_qd_0e6fe : Constant  Value=x_qd
  Constant_x_qd_49a0f : Constant  Value=x_qd
  Constant_x_qd_5f66a : Constant  Value=x_qd
  Constant_x_qdd_8ca24 : Constant  Value=x_qdd
  Constant_x_qdd_9ebba : Constant  Value=x_qdd
  Constant_x_qdd_d634e : Constant  Value=x_qdd
  Divide_1efda : Product  Inputs=*/
  Divide_217e1 : Product  Inputs=*/
  Divide_26786 : Product  Inputs=*/
  Divide_5ef35 : Product  Inputs=*/
  Divide_c3529 : Product  Inputs=*/
  Divide_cf3f8 : Product  Inputs=*/
  Product_0972b : Product
  Product_14059 : Product
  Product_19007 : Product
  Product_1ccbc : Product
  Product_440c4 : Product
  Product_4f485 : Product
  Product_74db8 : Product
  Product_798b6 : Product
  Product_8d60f : Product
  Product_a7861 : Product
  Product_dbeb6 : Product
  Subtract_0aeee : Sum  Inputs=+-
  Subtract_9c9ae : Sum  Inputs=+-
  Subtract_c835c : Sum  Inputs=+-
  Subtract_d5cbb : Sum  Inputs=+-
  Subtract_e222b : Sum  Inputs=+-
  Subtract_ec6e6 : Sum  Inputs=+-
  Subtract_ff27b : Sum  Inputs=+-
  Blockout_T_e_SG_D_3_1d3ff : Outport
  wires:
  State_psi_q_SG_D_3_76dcc/1 -> Add_41f88/2
  Constant_-1_0749c/1 -> Product_14059/1
  Subtract_e222b/1 -> Product_4f485/2
  State_psi_1d_SG_D_3_ba052/1 -> Product_a7861/2
  Constant_-1_d378a/1 -> Product_0972b/1
  Constant_x_l_08ff2/1 -> Product_0972b/2
  Add_1f3c8/1 -> Subtract_e222b/1
  State_psi_d_SG_D_3_65d7f/1 -> Add_1f3c8/2
  Product_0972b/1 -> Add_84477/1
  Constant_x_qdd_8ca24/1 -> Subtract_d5cbb/2
  Add_41f88/1 -> Product_8d60f/2
  Constant_x_qdd_9ebba/1 -> Add_84477/2
  State_psi_q_SG_D_3_c10b9/1 -> Product_4f485/1
  Constant_x_l_6d679/1 -> Product_14059/2
  Subtract_ff27b/1 -> Divide_cf3f8/2
  Constant_x_l_086ea/1 -> Subtract_c835c/2
  Constant_x_qd_0e6fe/1 -> Subtract_d5cbb/1
  Constant_-1_47889/1 -> Product_19007/1
  Subtract_0aeee/1 -> Divide_26786/2
  Constant_x_l_bb8da/1 -> Product_19007/2
  Product_798b6/1 -> Divide_26786/1
  Constant_-1_bd1df/1 -> Product_a7861/1
  Product_a7861/1 -> Product_798b6/1
  Constant_x_dd_4d15d/1 -> Subtract_9c9ae/1
  Constant_x_ddd_e3129/1 -> Subtract_9c9ae/2
  Add_0f122/1 -> Blockout_T_e_SG_D_3_1d3ff/1
  State_psi_gq_SG_D_3_42e3f/1 -> Product_440c4/1
  Product_4f485/1 -> Divide_c3529/1
  Add_84477/1 -> Product_440c4/2
  State_psi_fd_SG_D_3_c97e9/1 -> Product_1ccbc/1
  Product_14059/1 -> Add_39479/1
  Constant_x_qd_5f66a/1 -> Add_39479/2
  Constant_x_dd_dddf6/1 -> Subtract_0aeee/1
  State_psi_kq_SG_D_3_2048a/1 -> Product_dbeb6/1
  Constant_x_dd_fdaa2/1 -> Subtract_ff27b/1
  Subtract_d5cbb/1 -> Product_dbeb6/2
  Product_8d60f/1 -> Divide_5ef35/1
  Product_19007/1 -> Add_42a7e/1
  Add_39479/1 -> Divide_1efda/2
  Constant_x_qd_49a0f/1 -> Add_42a7e/2
  Subtract_9c9ae/1 -> Product_798b6/2
  Constant_x_l_b235b/1 -> Subtract_0aeee/2
  Constant_x_ddd_39604/1 -> Subtract_c835c/1
  Product_440c4/1 -> Divide_1efda/1
  Product_dbeb6/1 -> Divide_217e1/1
  Add_42a7e/1 -> Divide_217e1/2
  Constant_x_ddd_592bf/1 -> Divide_c3529/2
  Subtract_c835c/1 -> Product_1ccbc/2
  Divide_1efda/1 -> Subtract_ec6e6/1
  Constant_x_l_26133/1 -> Subtract_ff27b/2
  Divide_217e1/1 -> Subtract_ec6e6/2
  Divide_26786/1 -> Add_1f3c8/1
  Product_1ccbc/1 -> Divide_cf3f8/1
  Constant_-1_25f76/1 -> Product_74db8/1
  State_psi_d_SG_D_3_1c144/1 -> Product_74db8/2
  Subtract_ec6e6/1 -> Add_41f88/1
  Divide_cf3f8/1 -> Subtract_e222b/2
  Product_74db8/1 -> Product_8d60f/1
  Constant_x_qdd_d634e/1 -> Divide_5ef35/2
  Divide_5ef35/1 -> Add_0f122/1
  Divide_c3529/1 -> Add_0f122/2

== system case3/SG_D_3/d_E_fd_SG_D_3_block ==
  note: d_E_fd_SG_D_3 in case3
      | $\frac{V_{f,\mathrm{SG},D,3}-E_{\mathrm{fd},\mathrm{SG},D,3}\,K_{E}}{T_{E}}$
      | Automatically generated on 2025-10-31 19:01:25 .
  State_E_fd_SG_D_3_7cd07 : Inport
  State_V_f_SG_D_3_40669 : Inport  Port=2
  Add_e658e : Sum
  Constant_-1_43c23 : Constant  Value=-1
  Constant_K_E_94686 : Constant  Value=K_E
  Constant_T_E_ef47a : Constant  Value=T_E
  Divide_a14d5 : Product  Inputs=*/
  Product_9da03 : Product
  Product_c4b64 : Product
  Blockout_d_E_fd_SG_D_3_8845a : Outport
  wires:
  State_V_f_SG_D_3_40669/1 -> Add_e658e/2
  Constant_-1_43c23/1 -> Product_c4b64/1
  State_E_fd_SG_D_3_7cd07/1 -> Product_c4b64/2
  Constant_T_E_ef47a/1 -> Divide_a14d5/2
  Product_c4b64/1 -> Product_9da03/1
  Product_9da03/1 -> Add_e658e/1
  Constant_K_E_94686/1 -> Product_9da03/2
  Divide_a14d5/1 -> Blockout_d_E_fd_SG_D_3_8845a/1
  Add_e658e/1 -> Divide_a14d5/1

== system case3/SG_D_3/d_Px_1_SG_D_3_block ==
  note: d_Px_1_SG_D_3 in case3
      | $\frac{w_{\mathrm{SG},D,3}-2\,\pi \,f_{0}}{T_{w}}-\frac{\mathrm{Px}_{1,\mathrm{SG},D,3}}{T_{w}}$
      | Automatically generated on 2025-10-31 19:01:26 .
  State_Px_1_SG_D_3_32a62 : Inport
  State_w_SG_D_3_a2340 : Inport  Port=2
  Add_d5f96 : Sum
  Add_dca72 : Sum
  Constant_-1_ccd99 : Constant  Value=-1
  Constant_-2.0_f7a0a : Constant  Value=-2.0
  Constant_T_w_23cad : Constant  Value=T_w
  Constant_T_w_c51f4 : Constant  Value=T_w
  Constant_f0_7af10 : Constant  Value=f0
  Constant_pi_e3c31 : Constant  Value=pi
  Divide_53d4e : Product  Inputs=*/
  Divide_e1cd5 : Product  Inputs=*/
  Product_43531 : Product
  Product_a7c1e : Product
  Product_e1a2f : Product
  Blockout_d_Px_1_SG_D_3_25376 : Outport
  wires:
  Constant_f0_7af10/1 -> Product_a7c1e/2
  Constant_-1_ccd99/1 -> Product_43531/1
  Constant_-2.0_f7a0a/1 -> Product_e1a2f/1
  Constant_pi_e3c31/1 -> Product_e1a2f/2
  Product_e1a2f/1 -> Product_a7c1e/1
  State_w_SG_D_3_a2340/1 -> Add_dca72/2
  Divide_e1cd5/1 -> Add_d5f96/1
  State_Px_1_SG_D_3_32a62/1 -> Product_43531/2
  Product_a7c1e/1 -> Add_dca72/1
  Product_43531/1 -> Divide_e1cd5/1
  Constant_T_w_c51f4/1 -> Divide_e1cd5/2
  Add_dca72/1 -> Divide_53d4e/1
  Constant_T_w_23cad/1 -> Divide_53d4e/2
  Divide_53d4e/1 -> Add_d5f96/2
  Add_d5f96/1 -> Blockout_d_Px_1_SG_D_3_25376/1

== system case3/SG_D_3/d_Px_2_SG_D_3_block ==
  note: d_Px_2_SG_D_3 in case3
      | $\frac{\mathrm{Px}_{1,\mathrm{SG},D,3}-T_{2}\,\left(\frac{\mathrm{Px}_{1,\mathrm{SG},D,3}}{T_{w}}-\frac{w_{\mathrm{SG},D,3}-2\,\pi \,f_{0}}{T_{w}}\right)}{T_{1}}-\frac{\mathrm{Px}_{2,\mathrm{SG},D,3}}{T_{1}}$
      | Automatically generated on 2025-10-31 19:01:28 .
  State_Px_2_SG_D_3_1f8e6 : Inport
  State_Px_1_SG_D_3_a5179 : Inport  Port=2
  State_Px_1_SG_D_3_97597 : Inport  Port=3
  State_w_SG_D_3_5fd48 : Inport  Port=4
  Add_83952 : Sum
  Add_e5a16 : Sum
  Add_e9a21 : Sum
  Add_f667f : Sum
  Constant_-1_33029 : Constant  Value=-1
  Constant_-1_60966 : Constant  Value=-1
  Constant_-2.0_fccc5 : Constant  Value=-2.0
  Constant_T_1_a9e5e : Constant  Value=T_1
  Constant_T_1_d227f : Constant  Value=T_1
  Constant_T_2_bb8c0 : Constant  Value=T_2
  Constant_T_w_586ed : Constant  Value=T_w
  Constant_T_w_b76e7 : Constant  Value=T_w
  Constant_f0_4c787 : Constant  Value=f0
  Constant_pi_864f9 : Constant  Value=pi
  Divide_4976c : Product  Inputs=*/
  Divide_ae826 : Product  Inputs=*/
  Divide_bf287 : Product  Inputs=*/
  Divide_ef66a : Product  Inputs=*/
  Product_099e9 : Product
  Product_31ac6 : Product
  Product_53f11 : Product
  Product_b549f : Product
  Product_ffeee : Product
  Blockout_d_Px_2_SG_D_3_2a6eb : Outport
  wires:
  State_Px_1_SG_D_3_97597/1 -> Product_b549f/2
  Constant_-2.0_fccc5/1 -> Product_31ac6/1
  Constant_f0_4c787/1 -> Product_53f11/2
  Constant_pi_864f9/1 -> Product_31ac6/2
  Product_31ac6/1 -> Product_53f11/1
  State_w_SG_D_3_5fd48/1 -> Add_e5a16/2
  Constant_-1_33029/1 -> Product_b549f/1
  Product_53f11/1 -> Add_e5a16/1
  Product_b549f/1 -> Divide_ae826/1
  Constant_T_w_586ed/1 -> Divide_ae826/2
  Add_e5a16/1 -> Divide_4976c/1
  Constant_T_w_b76e7/1 -> Divide_4976c/2
  Divide_ae826/1 -> Add_f667f/1
  Divide_4976c/1 -> Add_f667f/2
  Constant_T_2_bb8c0/1 -> Product_099e9/1
  Add_f667f/1 -> Product_099e9/2
  Constant_-1_60966/1 -> Product_ffeee/1
  Product_099e9/1 -> Add_83952/2
  State_Px_2_SG_D_3_1f8e6/1 -> Product_ffeee/2
  State_Px_1_SG_D_3_a5179/1 -> Add_83952/1
  Product_ffeee/1 -> Divide_bf287/1
  Add_e9a21/1 -> Blockout_d_Px_2_SG_D_3_2a6eb/1
  Constant_T_1_d227f/1 -> Divide_bf287/2
  Add_83952/1 -> Divide_ef66a/1
  Constant_T_1_a9e5e/1 -> Divide_ef66a/2
  Divide_bf287/1 -> Add_e9a21/1
  Divide_ef66a/1 -> Add_e9a21/2

== system case3/SG_D_3/d_Px_3_SG_D_3_block ==
  note: d_Px_3_SG_D_3 in case3
      | $\frac{\mathrm{Px}_{2,\mathrm{SG},D,3}+T_{4}\,\left(\frac{\mathrm{Px}_{1,\mathrm{SG},D,3}-T_{2}\,\left(\frac{\mathrm{Px}_{1,\mathrm{SG},D,3}}{T_{w}}-\frac{w_{\mathrm{SG},D,3}-2\,\pi \,f_{0}}{T_{w}}\right)}{T_{1}}-\frac{\mathrm{Px}_{2,\mathrm{SG},D,3}}{T_{1}}\right)}{T_{3}}-\frac{\mathrm{Px}_{3,\mathrm{SG},D,3}}{T_{3}}$
      | Automatically generated on 2025-10-31 19:01:30 .
  State_Px_3_SG_D_3_77d5b : Inport
  State_Px_2_SG_D_3_e9479 : Inport  Port=2
  State_Px_2_SG_D_3_1a96a : Inport  Port=3
  State_Px_1_SG_D_3_d42a9 : Inport  Port=4
  State_Px_1_SG_D_3_54980 : Inport  Port=5
  State_w_SG_D_3_1436e : Inport  Port=6
  Add_18518 : Sum
  Add_32d8c : Sum
  Add_450ff : Sum
  Add_b7fc2 : Sum
  Add_c903b : Sum
  Add_dcf37 : Sum
  Constant_-1_6cdc8 : Constant  Value=-1
  Constant_-1_907d9 : Constant  Value=-1
  Constant_-1_aa919 : Constant  Value=-1
  Constant_-2.0_7b919 : Constant  Value=-2.0
  Constant_T_1_b19f2 : Constant  Value=T_1
  Constant_T_1_e2516 : Constant  Value=T_1
  Constant_T_2_11b15 : Constant  Value=T_2
  Constant_T_3_2b959 : Constant  Value=T_3
  Constant_T_3_31bc8 : Constant  Value=T_3
  Constant_T_4_09b23 : Constant  Value=T_4
  Constant_T_w_6783a : Constant  Value=T_w
  Constant_T_w_dc0da : Constant  Value=T_w
  Constant_f0_cbfce : Constant  Value=f0
  Constant_pi_c9d5d : Constant  Value=pi
  Divide_3036c : Product  Inputs=*/
  Divide_5f0a0 : Product  Inputs=*/
  Divide_6830d : Product  Inputs=*/
  Divide_846df : Product  Inputs=*/
  Divide_9097f : Product  Inputs=*/
  Divide_d8e76 : Product  Inputs=*/
  Product_1b664 : Product
  Product_23c5a : Product
  Product_36548 : Product
  Product_3ef62 : Product
  Product_46478 : Product
  Product_8f5dd : Product
  Product_95a41 : Product
  Blockout_d_Px_3_SG_D_3_0e541 : Outport
  wires:
  State_Px_1_SG_D_3_54980/1 -> Product_36548/2
  Constant_f0_cbfce/1 -> Product_46478/2
  Constant_-2.0_7b919/1 -> Product_3ef62/1
  Add_b7fc2/1 -> Divide_9097f/1
  Constant_pi_c9d5d/1 -> Product_3ef62/2
  Product_3ef62/1 -> Product_46478/1
  State_w_SG_D_3_1436e/1 -> Add_dcf37/2
  Constant_T_w_6783a/1 -> Divide_3036c/2
  Constant_-1_907d9/1 -> Product_36548/1
  Product_46478/1 -> Add_dcf37/1
  Product_36548/1 -> Divide_3036c/1
  Add_dcf37/1 -> Divide_846df/1
  Product_1b664/1 -> Divide_6830d/1
  Constant_T_w_dc0da/1 -> Divide_846df/2
  Divide_3036c/1 -> Add_c903b/1
  Divide_846df/1 -> Add_c903b/2
  Constant_T_2_11b15/1 -> Product_23c5a/1
  Add_c903b/1 -> Product_23c5a/2
  Constant_-1_aa919/1 -> Product_1b664/1
  State_Px_2_SG_D_3_1a96a/1 -> Product_1b664/2
  State_Px_1_SG_D_3_d42a9/1 -> Add_b7fc2/1
  Constant_T_3_2b959/1 -> Divide_5f0a0/2
  Product_23c5a/1 -> Add_b7fc2/2
  Constant_T_1_e2516/1 -> Divide_6830d/2
  Add_450ff/1 -> Product_8f5dd/2
  Constant_T_1_b19f2/1 -> Divide_9097f/2
  Divide_d8e76/1 -> Add_32d8c/2
  Divide_6830d/1 -> Add_450ff/1
  Divide_9097f/1 -> Add_450ff/2
  Constant_T_4_09b23/1 -> Product_8f5dd/1
  Constant_-1_6cdc8/1 -> Product_95a41/1
  State_Px_3_SG_D_3_77d5b/1 -> Product_95a41/2
  State_Px_2_SG_D_3_e9479/1 -> Add_18518/1
  Product_8f5dd/1 -> Add_18518/2
  Product_95a41/1 -> Divide_5f0a0/1
  Add_18518/1 -> Divide_d8e76/1
  Constant_T_3_31bc8/1 -> Divide_d8e76/2
  Divide_5f0a0/1 -> Add_32d8c/1
  Add_32d8c/1 -> Blockout_d_Px_3_SG_D_3_0e541/1
